simulink model "MobileSimulator"  (R2020a)
settings: Solver=FixedStepAuto  StartTime=0.0  StopTime=5  FixedStep=0.0001  MaxStep=0.1  RelTol=1e-3
undefined symbols (not defined in the file): rad, s
libraries: simulink x7, aerolibconvert2 x4
settings Model: Creator=DELL  LastModifiedBy=DELL

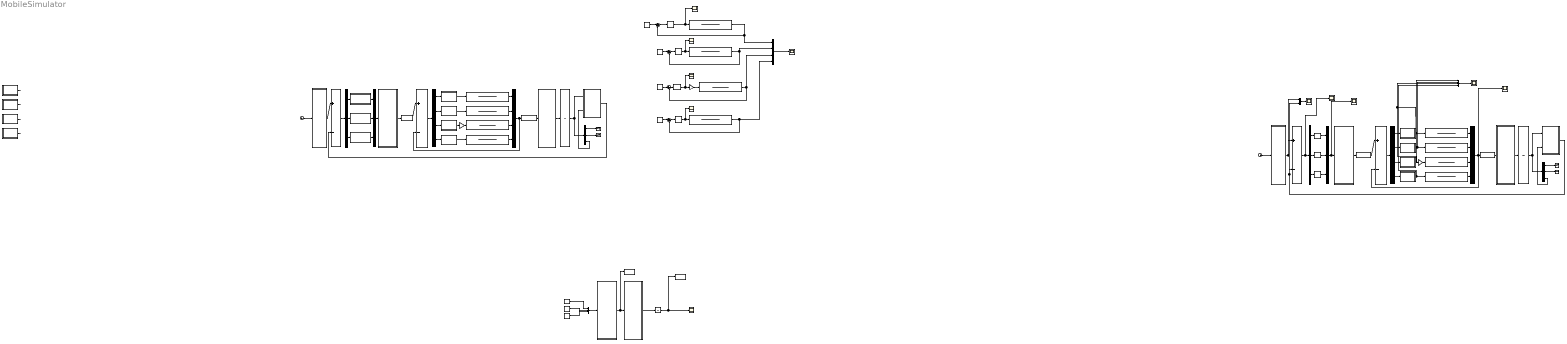
== system MobileSimulator ==
  note: Position Controller
  note: Velocity Controller
  note: Position Controller
  note: Velocity Controller
  Angular Velocity Conversion : aerolibconvert2/Angular Velocity Conversion  IU=rad/s  OU=rpm
  Angular Velocity Conversion1 : aerolibconvert2/Angular Velocity Conversion  IU=rpm  OU=rad/s
  Angular Velocity Conversion2 : aerolibconvert2/Angular Velocity Conversion  IU=rad/s  OU=rpm
  Angular Velocity Conversion3 : aerolibconvert2/Angular Velocity Conversion  IU=rpm  OU=rad/s
  Clock : Clock
  Clock1 : Clock
  Constant{,1..3} (4 alike) : Constant  Value=320
  Constant4 : Constant
  Constant5 : Constant
  Constant6 : Constant  Value=0
  Demux : Demux
  Demux{1,3..4,11} (4 alike) : Demux  Outputs=3
  Demux2 : Demux
  DesiresTrajectory : MATLAB Function  TreatAsAtomicUnit=on
  DesiresTrajectory1 : MATLAB Function  TreatAsAtomicUnit=on
  DriverMotor_1 : TransferFcn  Numerator=[6226000]  Denominator=[1 17030 178900]
  DriverMotor_10 : TransferFcn  Numerator=[6500000]  Denominator=[1 17520 180300]
  DriverMotor_11 : TransferFcn  Numerator=[1081000]  Denominator=[1 4692 40510]
  DriverMotor_12 : TransferFcn  Numerator=[7418000]  Denominator=[1 19890 214900]
  DriverMotor_2 : TransferFcn  Numerator=[6500000]  Denominator=[1 17520 180300]
  DriverMotor_3 : TransferFcn  Numerator=[1081000]  Denominator=[1 4692 40510]
  DriverMotor_4 : TransferFcn  Numerator=[7418000]  Denominator=[1 19890 214900]
  DriverMotor_5 : TransferFcn  Numerator=[6500000]  Denominator=[1 17520 180300]
  DriverMotor_6 : TransferFcn  Numerator=[6226000]  Denominator=[1 17030 178900]
  DriverMotor_7 : TransferFcn  Numerator=[1081000]  Denominator=[1 4692 40510]
  DriverMotor_8 : TransferFcn  Numerator=[7418000]  Denominator=[1 19890 214900]
  DriverMotor_9 : TransferFcn  Numerator=[6226000]  Denominator=[1 17030 178900]
  ForwardKinematic : MATLAB Function  TreatAsAtomicUnit=on
  ForwardKinematic1 : MATLAB Function  TreatAsAtomicUnit=on
  ForwardKinematic2 : MATLAB Function  TreatAsAtomicUnit=on
  Gain1 : Gain  Gain=1.3
  Gain2 : Gain  Gain=1.3
  Gain3 : Gain  Gain=1.3
  Integral : Integrator
  Integral1 : Integrator
  Integrator : Integrator
  InverseKinematics1 : MATLAB Function  TreatAsAtomicUnit=on
  InverseKinematics2 : MATLAB Function  TreatAsAtomicUnit=on
  InverseKinematics3 : MATLAB Function  TreatAsAtomicUnit=on
  Mux{,1,4,12} (4 alike) : Mux
  Mux2 : Mux  Inputs=3
  Mux3 : Mux  Inputs=3
  Mux5 : Mux  Inputs=3
  Mux6 : Mux  Inputs=2
  PDTheta : Subsystem
  PDX : Subsystem
  PDY : Subsystem
  PID Controller10 : simulink/Continuous/PID Controller  Controller=PI  Form=Parallel  TimeDomain=Continuous-time  UseExternalTs=off  SampleTime=-1  IntegratorMethod=Forward Euler  FilterMethod=Forward Euler  ControllerParametersSource=internal  P=0.460464335792483  I=15.4926513743787  D=0  UseFilter=on  N=100  TunerSelectOption=Transfer Function Based (PID Tuner App)  InitialConditionSource=internal  InitialConditionForIntegrator=0  InitialConditionForFilter=0  DifferentiatorICPrevScaledInput=0  ExternalReset=none  TrackingMode=off  Kt=1  LimitOutput=on  UpperSaturationLimit=24  LowerSaturationLimit=-24  LinearizeAsGain=on  AntiWindupMode=none  Kb=1  POutMin=[]  POutMax=[]  IOutMin=[]  IOutMax=[]  DOutMin=[]  DOutMax=[]  NOutMin=[]  NOutMax=[]  SumOutMin=[]  SumOutMax=[]  SaturationOutMin=[]  SaturationOutMax=[]  PParamMin=[]  PParamMax=[]  IParamMin=[]  IParamMax=[]  DParamMin=[]  DParamMax=[]  NParamMin=[]  NParamMax=[]  KbParamMin=[]  KbParamMax=[]  KtParamMin=[]  KtParamMax=[]  KbOutMin=[]  KbOutMax=[]  KtOutMin=[]  KtOutMax=[]  IntegratorOutMin=[]  IntegratorOutMax=[]  FilterOutMin=[]  FilterOutMax=[]  SumI1OutMin=[]  SumI1OutMax=[]  SumI2OutMin=[]  SumI2OutMax=[]  SumI3OutMin=[]  SumI3OutMax=[]  SumI4OutMin=[]  SumI4OutMax=[]  SumDOutMin=[]  SumDOutMax=[]  DifferentiatorOutMin=[]  DifferentiatorOutMax=[]  FilterDiffOutCoefMin=[]  FilterDiffOutCoefMax=[]  ReciprocalOutMin=[]  ReciprocalOutMax=[]  SumDenOutMin=[]  SumDenOutMax=[]  SumNumOutMin=[]  SumNumOutMax=[]  DivideOutMin=[]  DivideOutMax=[]  UdiffTsProdOutMin=[]  UdiffTsProdOutMax=[]  NTsProdOutMin=[]  NTsProdOutMax=[]  UintegralTsProdOutMin=[]  UintegralTsProdOutMax=[]  UngainTsProdOutMin=[]  UngainTsProdOutMax=[]  IntegratorContinuousStateAttributes=''  IntegratorStateMustResolveToSignalObject=off  IntegratorRTWStateStorageClass=Auto  FilterContinuousStateAttributes=''  FilterStateMustResolveToSignalObject=off  FilterRTWStateStorageClass=Auto  ParallelPVariant=InternalParameters  IdealPVariant=Disabled  IVariant=InternalParameters  DVariant=Disabled  IntegratorVariant=Continuous  SatVariant=Enabled  AWVariant=Passthrough  PCopyVariant=Disabled  TRVariant=Disabled  FdbkBlocksVariant=Forward  IdealPFdbkVariant=Disabled  SatFdbkVariant=Disabled  DerivativeFilterVariant=Disabled  NVariant=Disabled  NCopyVariant=Disabled_SignalSpec  FilterICVariant=Disabled  IntegratorICVariant=InternalICs  ExternalResetVariant=Disabled  TRSumVariant=Passthrough  SumFdbkVariant=Disabled  SumVariant=Sum_PI  TsampFilterVariant=InternalTs  TsampNgainVariant=Passthrough  TsampIntegralVariant=Passthrough
  PID Controller4 : simulink/Continuous/PID Controller  Controller=PD  Form=Parallel  TimeDomain=Continuous-time  UseExternalTs=off  SampleTime=-1  IntegratorMethod=Forward Euler  FilterMethod=Forward Euler  ControllerParametersSource=internal  P=31.494456693384  I=1403.5644395001  D=0  UseFilter=on  N=100  TunerSelectOption=Transfer Function Based (PID Tuner App)  InitialConditionSource=internal  InitialConditionForIntegrator=0  InitialConditionForFilter=0  DifferentiatorICPrevScaledInput=0  ExternalReset=none  TrackingMode=off  Kt=1  LimitOutput=on  UpperSaturationLimit=1  LowerSaturationLimit=-1  LinearizeAsGain=on  AntiWindupMode=none  Kb=1  POutMin=[]  POutMax=[]  IOutMin=[]  IOutMax=[]  DOutMin=[]  DOutMax=[]  NOutMin=[]  NOutMax=[]  SumOutMin=[]  SumOutMax=[]  SaturationOutMin=[]  SaturationOutMax=[]  PParamMin=[]  PParamMax=[]  IParamMin=[]  IParamMax=[]  DParamMin=[]  DParamMax=[]  NParamMin=[]  NParamMax=[]  KbParamMin=[]  KbParamMax=[]  KtParamMin=[]  KtParamMax=[]  KbOutMin=[]  KbOutMax=[]  KtOutMin=[]  KtOutMax=[]  IntegratorOutMin=[]  IntegratorOutMax=[]  FilterOutMin=[]  FilterOutMax=[]  SumI1OutMin=[]  SumI1OutMax=[]  SumI2OutMin=[]  SumI2OutMax=[]  SumI3OutMin=[]  SumI3OutMax=[]  SumI4OutMin=[]  SumI4OutMax=[]  SumDOutMin=[]  SumDOutMax=[]  DifferentiatorOutMin=[]  DifferentiatorOutMax=[]  FilterDiffOutCoefMin=[]  FilterDiffOutCoefMax=[]  ReciprocalOutMin=[]  ReciprocalOutMax=[]  SumDenOutMin=[]  SumDenOutMax=[]  SumNumOutMin=[]  SumNumOutMax=[]  DivideOutMin=[]  DivideOutMax=[]  UdiffTsProdOutMin=[]  UdiffTsProdOutMax=[]  NTsProdOutMin=[]  NTsProdOutMax=[]  UintegralTsProdOutMin=[]  UintegralTsProdOutMax=[]  UngainTsProdOutMin=[]  UngainTsProdOutMax=[]  IntegratorContinuousStateAttributes=''  IntegratorStateMustResolveToSignalObject=off  IntegratorRTWStateStorageClass=Auto  FilterContinuousStateAttributes=''  FilterStateMustResolveToSignalObject=off  FilterRTWStateStorageClass=Auto  ParallelPVariant=InternalParameters  IdealPVariant=Disabled  IVariant=Disabled  DVariant=InternalParameters  IntegratorVariant=Disabled  SatVariant=Enabled  AWVariant=Disabled  PCopyVariant=Disabled  TRVariant=Disabled  FdbkBlocksVariant=Forward  IdealPFdbkVariant=Disabled  SatFdbkVariant=Disabled  DerivativeFilterVariant=ContFilter  NVariant=InternalParameters  NCopyVariant=Disabled  FilterICVariant=InternalICsFilter  IntegratorICVariant=Disabled  ExternalResetVariant=Disabled  TRSumVariant=Passthrough  SumFdbkVariant=Disabled  SumVariant=Sum_PD  TsampFilterVariant=InternalTs  TsampNgainVariant=Passthrough  TsampIntegralVariant=Disabled_SignalSpec
  PID Controller5 : simulink/Continuous/PID Controller  Controller=PD  Form=Parallel  TimeDomain=Continuous-time  UseExternalTs=off  SampleTime=-1  IntegratorMethod=Forward Euler  FilterMethod=Forward Euler  ControllerParametersSource=internal  P=12.3118231803941  I=1  D=0  UseFilter=on  N=100  TunerSelectOption=Transfer Function Based (PID Tuner App)  InitialConditionSource=internal  InitialConditionForIntegrator=0  InitialConditionForFilter=0  DifferentiatorICPrevScaledInput=0  ExternalReset=none  TrackingMode=off  Kt=1  LimitOutput=on  UpperSaturationLimit=1  LowerSaturationLimit=-1  LinearizeAsGain=off  AntiWindupMode=none  Kb=1  POutMin=[]  POutMax=[]  IOutMin=[]  IOutMax=[]  DOutMin=[]  DOutMax=[]  NOutMin=[]  NOutMax=[]  SumOutMin=[]  SumOutMax=[]  SaturationOutMin=[]  SaturationOutMax=[]  PParamMin=[]  PParamMax=[]  IParamMin=[]  IParamMax=[]  DParamMin=[]  DParamMax=[]  NParamMin=[]  NParamMax=[]  KbParamMin=[]  KbParamMax=[]  KtParamMin=[]  KtParamMax=[]  KbOutMin=[]  KbOutMax=[]  KtOutMin=[]  KtOutMax=[]  IntegratorOutMin=[]  IntegratorOutMax=[]  FilterOutMin=[]  FilterOutMax=[]  SumI1OutMin=[]  SumI1OutMax=[]  SumI2OutMin=[]  SumI2OutMax=[]  SumI3OutMin=[]  SumI3OutMax=[]  SumI4OutMin=[]  SumI4OutMax=[]  SumDOutMin=[]  SumDOutMax=[]  DifferentiatorOutMin=[]  DifferentiatorOutMax=[]  FilterDiffOutCoefMin=[]  FilterDiffOutCoefMax=[]  ReciprocalOutMin=[]  ReciprocalOutMax=[]  SumDenOutMin=[]  SumDenOutMax=[]  SumNumOutMin=[]  SumNumOutMax=[]  DivideOutMin=[]  DivideOutMax=[]  UdiffTsProdOutMin=[]  UdiffTsProdOutMax=[]  NTsProdOutMin=[]  NTsProdOutMax=[]  UintegralTsProdOutMin=[]  UintegralTsProdOutMax=[]  UngainTsProdOutMin=[]  UngainTsProdOutMax=[]  IntegratorContinuousStateAttributes=''  IntegratorStateMustResolveToSignalObject=off  IntegratorRTWStateStorageClass=Auto  FilterContinuousStateAttributes=''  FilterStateMustResolveToSignalObject=off  FilterRTWStateStorageClass=Auto  ParallelPVariant=InternalParameters  IdealPVariant=Disabled  IVariant=Disabled  DVariant=InternalParameters  IntegratorVariant=Disabled  SatVariant=Enabled  AWVariant=Disabled  PCopyVariant=Disabled  TRVariant=Disabled  FdbkBlocksVariant=Forward  IdealPFdbkVariant=Disabled  SatFdbkVariant=Disabled  DerivativeFilterVariant=ContFilter  NVariant=InternalParameters  NCopyVariant=Disabled  FilterICVariant=InternalICsFilter  IntegratorICVariant=Disabled  ExternalResetVariant=Disabled  TRSumVariant=Passthrough  SumFdbkVariant=Disabled  SumVariant=Sum_PD  TsampFilterVariant=InternalTs  TsampNgainVariant=Passthrough  TsampIntegralVariant=Disabled_SignalSpec
  PID Controller6 : simulink/Continuous/PID Controller  Controller=PD  Form=Parallel  TimeDomain=Continuous-time  UseExternalTs=off  SampleTime=-1  IntegratorMethod=Forward Euler  FilterMethod=Forward Euler  ControllerParametersSource=internal  P=17.283663240322  I=1  D=0  UseFilter=on  N=100  TunerSelectOption=Transfer Function Based (PID Tuner App)  InitialConditionSource=internal  InitialConditionForIntegrator=0  InitialConditionForFilter=0  DifferentiatorICPrevScaledInput=0  ExternalReset=none  TrackingMode=off  Kt=1  LimitOutput=on  UpperSaturationLimit=1  LowerSaturationLimit=-1  LinearizeAsGain=on  AntiWindupMode=none  Kb=1  POutMin=[]  POutMax=[]  IOutMin=[]  IOutMax=[]  DOutMin=[]  DOutMax=[]  NOutMin=[]  NOutMax=[]  SumOutMin=[]  SumOutMax=[]  SaturationOutMin=[]  SaturationOutMax=[]  PParamMin=[]  PParamMax=[]  IParamMin=[]  IParamMax=[]  DParamMin=[]  DParamMax=[]  NParamMin=[]  NParamMax=[]  KbParamMin=[]  KbParamMax=[]  KtParamMin=[]  KtParamMax=[]  KbOutMin=[]  KbOutMax=[]  KtOutMin=[]  KtOutMax=[]  IntegratorOutMin=[]  IntegratorOutMax=[]  FilterOutMin=[]  FilterOutMax=[]  SumI1OutMin=[]  SumI1OutMax=[]  SumI2OutMin=[]  SumI2OutMax=[]  SumI3OutMin=[]  SumI3OutMax=[]  SumI4OutMin=[]  SumI4OutMax=[]  SumDOutMin=[]  SumDOutMax=[]  DifferentiatorOutMin=[]  DifferentiatorOutMax=[]  FilterDiffOutCoefMin=[]  FilterDiffOutCoefMax=[]  ReciprocalOutMin=[]  ReciprocalOutMax=[]  SumDenOutMin=[]  SumDenOutMax=[]  SumNumOutMin=[]  SumNumOutMax=[]  DivideOutMin=[]  DivideOutMax=[]  UdiffTsProdOutMin=[]  UdiffTsProdOutMax=[]  NTsProdOutMin=[]  NTsProdOutMax=[]  UintegralTsProdOutMin=[]  UintegralTsProdOutMax=[]  UngainTsProdOutMin=[]  UngainTsProdOutMax=[]  IntegratorContinuousStateAttributes=''  IntegratorStateMustResolveToSignalObject=off  IntegratorRTWStateStorageClass=Auto  FilterContinuousStateAttributes=''  FilterStateMustResolveToSignalObject=off  FilterRTWStateStorageClass=Auto  ParallelPVariant=InternalParameters  IdealPVariant=Disabled  IVariant=Disabled  DVariant=InternalParameters  IntegratorVariant=Disabled  SatVariant=Enabled  AWVariant=Disabled  PCopyVariant=Disabled  TRVariant=Disabled  FdbkBlocksVariant=Forward  IdealPFdbkVariant=Disabled  SatFdbkVariant=Disabled  DerivativeFilterVariant=ContFilter  NVariant=InternalParameters  NCopyVariant=Disabled  FilterICVariant=InternalICsFilter  IntegratorICVariant=Disabled  ExternalResetVariant=Disabled  TRSumVariant=Passthrough  SumFdbkVariant=Disabled  SumVariant=Sum_PD  TsampFilterVariant=InternalTs  TsampNgainVariant=Passthrough  TsampIntegralVariant=Disabled_SignalSpec
  PID Controller7 : simulink/Continuous/PID Controller  Controller=PI  Form=Parallel  TimeDomain=Continuous-time  UseExternalTs=off  SampleTime=-1  IntegratorMethod=Forward Euler  FilterMethod=Forward Euler  ControllerParametersSource=internal  P=0.460464335792483  I=15.4926513743787  D=0  UseFilter=on  N=100  TunerSelectOption=Transfer Function Based (PID Tuner App)  InitialConditionSource=internal  InitialConditionForIntegrator=0  InitialConditionForFilter=0  DifferentiatorICPrevScaledInput=0  ExternalReset=none  TrackingMode=off  Kt=1  LimitOutput=on  UpperSaturationLimit=24  LowerSaturationLimit=-24  LinearizeAsGain=on  AntiWindupMode=none  Kb=1  POutMin=[]  POutMax=[]  IOutMin=[]  IOutMax=[]  DOutMin=[]  DOutMax=[]  NOutMin=[]  NOutMax=[]  SumOutMin=[]  SumOutMax=[]  SaturationOutMin=[]  SaturationOutMax=[]  PParamMin=[]  PParamMax=[]  IParamMin=[]  IParamMax=[]  DParamMin=[]  DParamMax=[]  NParamMin=[]  NParamMax=[]  KbParamMin=[]  KbParamMax=[]  KtParamMin=[]  KtParamMax=[]  KbOutMin=[]  KbOutMax=[]  KtOutMin=[]  KtOutMax=[]  IntegratorOutMin=[]  IntegratorOutMax=[]  FilterOutMin=[]  FilterOutMax=[]  SumI1OutMin=[]  SumI1OutMax=[]  SumI2OutMin=[]  SumI2OutMax=[]  SumI3OutMin=[]  SumI3OutMax=[]  SumI4OutMin=[]  SumI4OutMax=[]  SumDOutMin=[]  SumDOutMax=[]  DifferentiatorOutMin=[]  DifferentiatorOutMax=[]  FilterDiffOutCoefMin=[]  FilterDiffOutCoefMax=[]  ReciprocalOutMin=[]  ReciprocalOutMax=[]  SumDenOutMin=[]  SumDenOutMax=[]  SumNumOutMin=[]  SumNumOutMax=[]  DivideOutMin=[]  DivideOutMax=[]  UdiffTsProdOutMin=[]  UdiffTsProdOutMax=[]  NTsProdOutMin=[]  NTsProdOutMax=[]  UintegralTsProdOutMin=[]  UintegralTsProdOutMax=[]  UngainTsProdOutMin=[]  UngainTsProdOutMax=[]  IntegratorContinuousStateAttributes=''  IntegratorStateMustResolveToSignalObject=off  IntegratorRTWStateStorageClass=Auto  FilterContinuousStateAttributes=''  FilterStateMustResolveToSignalObject=off  FilterRTWStateStorageClass=Auto  ParallelPVariant=InternalParameters  IdealPVariant=Disabled  IVariant=InternalParameters  DVariant=Disabled  IntegratorVariant=Continuous  SatVariant=Enabled  AWVariant=Passthrough  PCopyVariant=Disabled  TRVariant=Disabled  FdbkBlocksVariant=Forward  IdealPFdbkVariant=Disabled  SatFdbkVariant=Disabled  DerivativeFilterVariant=Disabled  NVariant=Disabled  NCopyVariant=Disabled_SignalSpec  FilterICVariant=Disabled  IntegratorICVariant=InternalICs  ExternalResetVariant=Disabled  TRSumVariant=Passthrough  SumFdbkVariant=Disabled  SumVariant=Sum_PI  TsampFilterVariant=InternalTs  TsampNgainVariant=Passthrough  TsampIntegralVariant=Passthrough
  PID Controller8 : simulink/Continuous/PID Controller  Controller=PI  Form=Parallel  TimeDomain=Continuous-time  UseExternalTs=off  SampleTime=-1  IntegratorMethod=Forward Euler  FilterMethod=Forward Euler  ControllerParametersSource=internal  P=0.460464335792483  I=15.4926513743787  D=0  UseFilter=on  N=100  TunerSelectOption=Transfer Function Based (PID Tuner App)  InitialConditionSource=internal  InitialConditionForIntegrator=0  InitialConditionForFilter=0  DifferentiatorICPrevScaledInput=0  ExternalReset=none  TrackingMode=off  Kt=1  LimitOutput=on  UpperSaturationLimit=24  LowerSaturationLimit=-24  LinearizeAsGain=on  AntiWindupMode=none  Kb=1  POutMin=[]  POutMax=[]  IOutMin=[]  IOutMax=[]  DOutMin=[]  DOutMax=[]  NOutMin=[]  NOutMax=[]  SumOutMin=[]  SumOutMax=[]  SaturationOutMin=[]  SaturationOutMax=[]  PParamMin=[]  PParamMax=[]  IParamMin=[]  IParamMax=[]  DParamMin=[]  DParamMax=[]  NParamMin=[]  NParamMax=[]  KbParamMin=[]  KbParamMax=[]  KtParamMin=[]  KtParamMax=[]  KbOutMin=[]  KbOutMax=[]  KtOutMin=[]  KtOutMax=[]  IntegratorOutMin=[]  IntegratorOutMax=[]  FilterOutMin=[]  FilterOutMax=[]  SumI1OutMin=[]  SumI1OutMax=[]  SumI2OutMin=[]  SumI2OutMax=[]  SumI3OutMin=[]  SumI3OutMax=[]  SumI4OutMin=[]  SumI4OutMax=[]  SumDOutMin=[]  SumDOutMax=[]  DifferentiatorOutMin=[]  DifferentiatorOutMax=[]  FilterDiffOutCoefMin=[]  FilterDiffOutCoefMax=[]  ReciprocalOutMin=[]  ReciprocalOutMax=[]  SumDenOutMin=[]  SumDenOutMax=[]  SumNumOutMin=[]  SumNumOutMax=[]  DivideOutMin=[]  DivideOutMax=[]  UdiffTsProdOutMin=[]  UdiffTsProdOutMax=[]  NTsProdOutMin=[]  NTsProdOutMax=[]  UintegralTsProdOutMin=[]  UintegralTsProdOutMax=[]  UngainTsProdOutMin=[]  UngainTsProdOutMax=[]  IntegratorContinuousStateAttributes=''  IntegratorStateMustResolveToSignalObject=off  IntegratorRTWStateStorageClass=Auto  FilterContinuousStateAttributes=''  FilterStateMustResolveToSignalObject=off  FilterRTWStateStorageClass=Auto  ParallelPVariant=InternalParameters  IdealPVariant=Disabled  IVariant=InternalParameters  DVariant=Disabled  IntegratorVariant=Continuous  SatVariant=Enabled  AWVariant=Passthrough  PCopyVariant=Disabled  TRVariant=Disabled  FdbkBlocksVariant=Forward  IdealPFdbkVariant=Disabled  SatFdbkVariant=Disabled  DerivativeFilterVariant=Disabled  NVariant=Disabled  NCopyVariant=Disabled_SignalSpec  FilterICVariant=Disabled  IntegratorICVariant=InternalICs  ExternalResetVariant=Disabled  TRSumVariant=Passthrough  SumFdbkVariant=Disabled  SumVariant=Sum_PI  TsampFilterVariant=InternalTs  TsampNgainVariant=Passthrough  TsampIntegralVariant=Passthrough
  PID Controller9 : simulink/Continuous/PID Controller  Controller=PI  Form=Parallel  TimeDomain=Continuous-time  UseExternalTs=off  SampleTime=-1  IntegratorMethod=Forward Euler  FilterMethod=Forward Euler  ControllerParametersSource=internal  P=0.537194587615843  I=14.0924173229999  D=0  UseFilter=on  N=100  TunerSelectOption=Transfer Function Based (PID Tuner App)  InitialConditionSource=internal  InitialConditionForIntegrator=0  InitialConditionForFilter=0  DifferentiatorICPrevScaledInput=0  ExternalReset=none  TrackingMode=off  Kt=1  LimitOutput=on  UpperSaturationLimit=24  LowerSaturationLimit=-24  LinearizeAsGain=on  AntiWindupMode=none  Kb=1  POutMin=[]  POutMax=[]  IOutMin=[]  IOutMax=[]  DOutMin=[]  DOutMax=[]  NOutMin=[]  NOutMax=[]  SumOutMin=[]  SumOutMax=[]  SaturationOutMin=[]  SaturationOutMax=[]  PParamMin=[]  PParamMax=[]  IParamMin=[]  IParamMax=[]  DParamMin=[]  DParamMax=[]  NParamMin=[]  NParamMax=[]  KbParamMin=[]  KbParamMax=[]  KtParamMin=[]  KtParamMax=[]  KbOutMin=[]  KbOutMax=[]  KtOutMin=[]  KtOutMax=[]  IntegratorOutMin=[]  IntegratorOutMax=[]  FilterOutMin=[]  FilterOutMax=[]  SumI1OutMin=[]  SumI1OutMax=[]  SumI2OutMin=[]  SumI2OutMax=[]  SumI3OutMin=[]  SumI3OutMax=[]  SumI4OutMin=[]  SumI4OutMax=[]  SumDOutMin=[]  SumDOutMax=[]  DifferentiatorOutMin=[]  DifferentiatorOutMax=[]  FilterDiffOutCoefMin=[]  FilterDiffOutCoefMax=[]  ReciprocalOutMin=[]  ReciprocalOutMax=[]  SumDenOutMin=[]  SumDenOutMax=[]  SumNumOutMin=[]  SumNumOutMax=[]  DivideOutMin=[]  DivideOutMax=[]  UdiffTsProdOutMin=[]  UdiffTsProdOutMax=[]  NTsProdOutMin=[]  NTsProdOutMax=[]  UintegralTsProdOutMin=[]  UintegralTsProdOutMax=[]  UngainTsProdOutMin=[]  UngainTsProdOutMax=[]  IntegratorContinuousStateAttributes=''  IntegratorStateMustResolveToSignalObject=off  IntegratorRTWStateStorageClass=Auto  FilterContinuousStateAttributes=''  FilterStateMustResolveToSignalObject=off  FilterRTWStateStorageClass=Auto  ParallelPVariant=InternalParameters  IdealPVariant=Disabled  IVariant=InternalParameters  DVariant=Disabled  IntegratorVariant=Continuous  SatVariant=Enabled  AWVariant=Passthrough  PCopyVariant=Disabled  TRVariant=Disabled  FdbkBlocksVariant=Forward  IdealPFdbkVariant=Disabled  SatFdbkVariant=Disabled  DerivativeFilterVariant=Disabled  NVariant=Disabled  NCopyVariant=Disabled_SignalSpec  FilterICVariant=Disabled  IntegratorICVariant=InternalICs  ExternalResetVariant=Disabled  TRSumVariant=Passthrough  SumFdbkVariant=Disabled  SumVariant=Sum_PI  TsampFilterVariant=InternalTs  TsampNgainVariant=Passthrough  TsampIntegralVariant=Passthrough
  PI_Motor_1. : Subsystem
  PI_Motor_10 : Subsystem
  PI_Motor_11 : Subsystem
  PI_Motor_12 : Subsystem
  PI_Motor_2. : Subsystem
  PI_Motor_3. : Subsystem
  PI_Motor_4. : Subsystem
  PI_Motor_5 : Subsystem
  PI_Motor_6 : Subsystem
  PI_Motor_7 : Subsystem
  PI_Motor_8 : Subsystem
  PI_Motor_9 : Subsystem
  Scope{,2..3,6..8,11,13..15,17} (11 alike) : Scope
  Sum{,1,3..6} (6 alike) : Sum  Inputs=|+-
  Sum. : Sum  Inputs=|+-
  Sum.1 : Sum  Inputs=|+-
  Terminator{1..2,6..7} (4 alike) : Terminator
  To File : ToFile  Filename=D:\Documents\DOAN\DO-AN\matlab\datamat\dothi\banhxe.mat
  To File1 : ToFile  Filename=D:\Documents\DOAN\DO-AN\matlab\datamat\dothi\vitri.mat
  ToGlobal : MATLAB Function  TreatAsAtomicUnit=on
  ToGlobal1 : MATLAB Function  TreatAsAtomicUnit=on
  wires:
  PI_Motor_1./1(signal) -> DriverMotor_1/1
  PI_Motor_2./1(signal) -> DriverMotor_2/1
  PI_Motor_4./1(signal) -> DriverMotor_4/1
  DriverMotor_1/1 -> Mux/1
  DriverMotor_2/1 -> Mux/2
  DriverMotor_4/1 -> Mux/4
  Demux/1 -> PI_Motor_1./1(error)
  Demux/2 -> PI_Motor_2./1(error)
  Demux/4 -> PI_Motor_4./1(error)
  Demux/3 -> PI_Motor_3./1(error)
  Sum/1 -> Demux/1
  InverseKinematics2/1(w) -> Angular Velocity Conversion/1
  ForwardKinematic/1(q_dot_r) -> Integral/1
  Sum./1 -> Demux1/1
  Integral/1 -> Demux11/1, ToGlobal/1(q_r)
  Demux11/1 -> Terminator6/1
  Demux11/2 -> Terminator7/1
  ToGlobal/1(q) -> Sum./2
  DesiresTrajectory/1(q) -> Sum./1
  Clock/1 -> DesiresTrajectory/1(t)
  Mux2/1 -> InverseKinematics2/1(q_dot_r)
  Demux11/3 -> ToGlobal/2(theta)
  Demux1/1 -> PDX/1(error)
  PDX/1(signal) -> Mux2/1
  Demux1/2 -> PDY/1(error)
  PDY/1(signal) -> Mux2/2
  Demux1/3 -> PDTheta/1(error)
  PDTheta/1(signal) -> Mux2/3
  Mux/1 -> Sum/2, Angular Velocity Conversion1/1
  Angular Velocity Conversion/1 -> Sum/1
  Angular Velocity Conversion1/1 -> ForwardKinematic/1(w)
  PID Controller8/1 -> Scope11/1, DriverMotor_5/1
  Sum3/1 -> PID Controller8/1
  PI_Motor_5/1(signal) -> ?
  PI_Motor_6/1(signal) -> ?
  PI_Motor_8/1(signal) -> ?
  PI_Motor_7/1(signal) -> ?
  Sum4/1 -> PID Controller7/1
  Constant3/1 -> Sum4/1
  Constant/1 -> Sum3/1
  DriverMotor_5/1 -> Mux12/2, Sum3/2
  PID Controller7/1 -> DriverMotor_6/1, Scope13/1
  DriverMotor_6/1 -> Sum4/2, Mux12/1
  Sum5/1 -> PID Controller9/1
  Constant1/1 -> Sum5/1
  Sum6/1 -> PID Controller10/1
  PID Controller10/1 -> DriverMotor_8/1, Scope17/1
  DriverMotor_8/1 -> Mux12/4, Sum6/2
  Constant2/1 -> Sum6/1
  DriverMotor_7/1 -> Mux12/3, Sum5/2
  Mux12/1 -> Scope14/1
  DriverMotor_3/1 -> Mux/3
  PID Controller9/1 -> Gain3/1, Scope15/1
  Gain1/1 -> DriverMotor_3/1
  Gain3/1 -> DriverMotor_7/1
  DriverMotor_12/1 -> Mux1/4
  Demux4/1 -> Terminator1/1
  PI_Motor_11/1(signal) -> DriverMotor_9/1, Mux4/1
  DriverMotor_10/1 -> Mux1/2
  Angular Velocity Conversion3/1 -> ForwardKinematic1/1(w)
  Demux3/2 -> PID Controller5/1
  Demux3/1 -> PID Controller4/1
  Demux3/3 -> PID Controller6/1
  PID Controller6/1 -> Mux5/3
  Mux6/1 -> Scope2/1
  Demux4/3 -> ToGlobal1/2(theta)
  PID Controller5/1 -> Mux5/2
  ToGlobal1/1(q) -> Mux6/2, Sum.1/2
  Mux5/1 -> InverseKinematics1/1(q_dot_r), Scope6/1
  Demux4/2 -> Terminator2/1
  Demux2/4 -> PI_Motor_9/1(error)
  PI_Motor_9/1(signal) -> DriverMotor_12/1, Mux4/4
  InverseKinematics1/1(w) -> Angular Velocity Conversion2/1
  Integral1/1 -> Demux4/1, ToGlobal1/1(q_r)
  Sum.1/1 -> Scope8/1, Demux3/1
  ForwardKinematic1/1(q_dot_r) -> Integral1/1
  PI_Motor_10/1(signal) -> Mux4/3, Gain2/1
  Sum1/1 -> Demux2/1
  DriverMotor_11/1 -> Mux1/3
  PI_Motor_12/1(signal) -> Mux4/2, DriverMotor_10/1
  Angular Velocity Conversion2/1 -> Sum1/1
  DriverMotor_9/1 -> Mux1/1
  Demux2/2 -> PI_Motor_12/1(error)
  DesiresTrajectory1/1(q) -> Mux6/1, Sum.1/1
  Mux4/1 -> Scope3/1
  Demux2/1 -> PI_Motor_11/1(error)
  PID Controller4/1 -> Mux5/1
  Clock1/1 -> DesiresTrajectory1/1(t)
  Gain2/1 -> DriverMotor_11/1
  Demux2/3 -> PI_Motor_10/1(error)
  Mux1/1 -> Sum1/2, Angular Velocity Conversion3/1, Scope7/1
  PI_Motor_3./1(signal) -> Gain1/1
  InverseKinematics3/1(w) -> To File/1, ForwardKinematic2/1(w)
  Mux3/1 -> InverseKinematics3/1(q_dot_r)
  Constant5/1 -> Mux3/2
  Constant4/1 -> Mux3/1
  Constant6/1 -> Mux3/3
  ForwardKinematic2/1(q_dot_r) -> Integrator/1
  Integrator/1 -> To File1/1, Scope/1

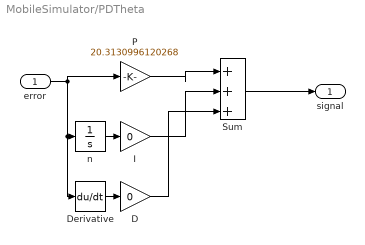
== system MobileSimulator/PDTheta ==
  error : Inport
  D : Gain  Gain=0
  Derivative : Derivative
  I : Gain  Gain=0
  P : Gain  Gain=20.3130996120268
  Sum : Sum  Inputs=|+++
  n : Integrator
  signal : Outport
  wires:
  Derivative/1 -> D/1
  n/1 -> I/1
  I/1 -> Sum/2
  error/1 -> Derivative/1, n/1, P/1
  Sum/1 -> signal/1
  P/1 -> Sum/1
  D/1 -> Sum/3

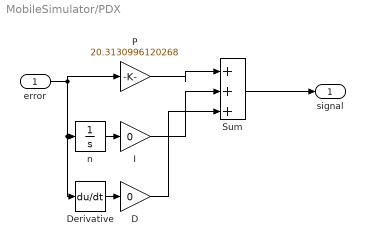
== system MobileSimulator/PDX ==
  error : Inport
  D : Gain  Gain=0
  Derivative : Derivative
  I : Gain  Gain=0
  P : Gain  Gain=20.3130996120268
  Sum : Sum  Inputs=|+++
  n : Integrator
  signal : Outport
  wires:
  Derivative/1 -> D/1
  n/1 -> I/1
  I/1 -> Sum/2
  error/1 -> Derivative/1, n/1, P/1
  Sum/1 -> signal/1
  P/1 -> Sum/1
  D/1 -> Sum/3

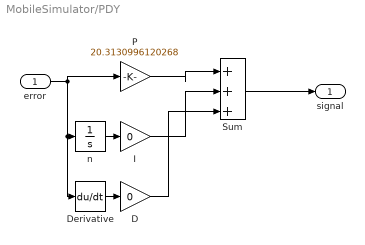
== system MobileSimulator/PDY ==
  error : Inport
  D : Gain  Gain=0
  Derivative : Derivative
  I : Gain  Gain=0
  P : Gain  Gain=20.3130996120268
  Sum : Sum  Inputs=|+++
  n : Integrator
  signal : Outport
  wires:
  Derivative/1 -> D/1
  n/1 -> I/1
  I/1 -> Sum/2
  error/1 -> Derivative/1, n/1, P/1
  Sum/1 -> signal/1
  P/1 -> Sum/1
  D/1 -> Sum/3

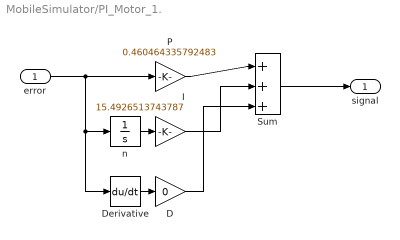
== system MobileSimulator/PI_Motor_1. ==
  error : Inport
  D : Gain  Gain=0
  Derivative : Derivative
  I : Gain  Gain=15.4926513743787
  P : Gain  Gain=0.460464335792483
  Sum : Sum  Inputs=|+++
  n : Integrator
  signal : Outport
  wires:
  error/1 -> P/1, n/1, Derivative/1
  n/1 -> I/1
  P/1 -> Sum/1
  I/1 -> Sum/2
  Derivative/1 -> D/1
  Sum/1 -> signal/1
  D/1 -> Sum/3

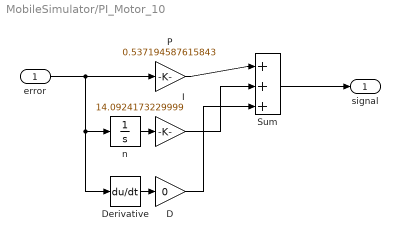
== system MobileSimulator/PI_Motor_10 ==
  error : Inport
  D : Gain  Gain=0
  Derivative : Derivative
  I : Gain  Gain=14.0924173229999
  P : Gain  Gain=0.537194587615843
  Sum : Sum  Inputs=|+++
  n : Integrator
  signal : Outport
  wires:
  Derivative/1 -> D/1
  n/1 -> I/1
  I/1 -> Sum/2
  error/1 -> P/1, n/1, Derivative/1
  Sum/1 -> signal/1
  P/1 -> Sum/1
  D/1 -> Sum/3

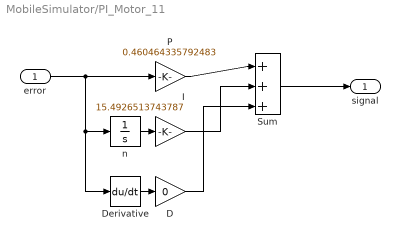
== system MobileSimulator/PI_Motor_11 ==
  error : Inport
  D : Gain  Gain=0
  Derivative : Derivative
  I : Gain  Gain=15.4926513743787
  P : Gain  Gain=0.460464335792483
  Sum : Sum  Inputs=|+++
  n : Integrator
  signal : Outport
  wires:
  error/1 -> P/1, n/1, Derivative/1
  n/1 -> I/1
  P/1 -> Sum/1
  I/1 -> Sum/2
  Derivative/1 -> D/1
  Sum/1 -> signal/1
  D/1 -> Sum/3

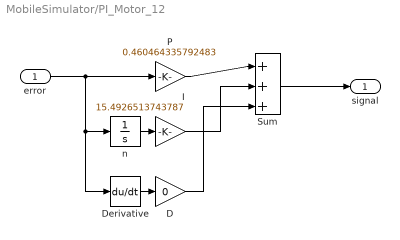
== system MobileSimulator/PI_Motor_12 ==
  error : Inport
  D : Gain  Gain=0
  Derivative : Derivative
  I : Gain  Gain=15.4926513743787
  P : Gain  Gain=0.460464335792483
  Sum : Sum  Inputs=|+++
  n : Integrator
  signal : Outport
  wires:
  error/1 -> P/1, n/1, Derivative/1
  n/1 -> I/1
  P/1 -> Sum/1
  I/1 -> Sum/2
  Derivative/1 -> D/1
  Sum/1 -> signal/1
  D/1 -> Sum/3

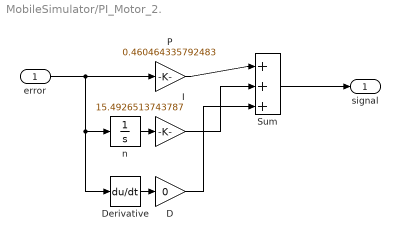
== system MobileSimulator/PI_Motor_2. ==
  error : Inport
  D : Gain  Gain=0
  Derivative : Derivative
  I : Gain  Gain=15.4926513743787
  P : Gain  Gain=0.460464335792483
  Sum : Sum  Inputs=|+++
  n : Integrator
  signal : Outport
  wires:
  error/1 -> P/1, n/1, Derivative/1
  n/1 -> I/1
  P/1 -> Sum/1
  I/1 -> Sum/2
  Derivative/1 -> D/1
  Sum/1 -> signal/1
  D/1 -> Sum/3

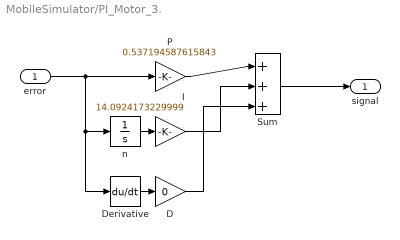
== system MobileSimulator/PI_Motor_3. ==
  error : Inport
  D : Gain  Gain=0
  Derivative : Derivative
  I : Gain  Gain=14.0924173229999
  P : Gain  Gain=0.537194587615843
  Sum : Sum  Inputs=|+++
  n : Integrator
  signal : Outport
  wires:
  Derivative/1 -> D/1
  n/1 -> I/1
  I/1 -> Sum/2
  error/1 -> P/1, n/1, Derivative/1
  Sum/1 -> signal/1
  P/1 -> Sum/1
  D/1 -> Sum/3

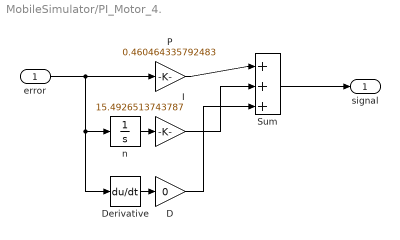
== system MobileSimulator/PI_Motor_4. ==
  error : Inport
  D : Gain  Gain=0
  Derivative : Derivative
  I : Gain  Gain=15.4926513743787
  P : Gain  Gain=0.460464335792483
  Sum : Sum  Inputs=|+++
  n : Integrator
  signal : Outport
  wires:
  error/1 -> P/1, n/1, Derivative/1
  n/1 -> I/1
  P/1 -> Sum/1
  I/1 -> Sum/2
  Derivative/1 -> D/1
  Sum/1 -> signal/1
  D/1 -> Sum/3

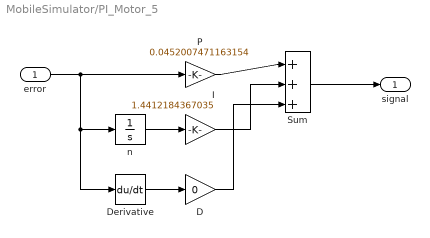
== system MobileSimulator/PI_Motor_5 ==
  error : Inport
  D : Gain  Gain=0
  Derivative : Derivative
  I : Gain  Gain=1.4412184367035
  P : Gain  Gain=0.0452007471163154
  Sum : Sum  Inputs=|+++
  n : Integrator
  signal : Outport
  wires:
  Derivative/1 -> D/1
  n/1 -> I/1
  I/1 -> Sum/2
  error/1 -> P/1, n/1, Derivative/1
  Sum/1 -> signal/1
  P/1 -> Sum/1
  D/1 -> Sum/3

== system MobileSimulator/PI_Motor_6 ==
  error : Inport
  D : Gain  Gain=0
  Derivative : Derivative
  I : Gain  Gain=1.79334556232624
  P : Gain  Gain=0.070850354012992
  Sum : Sum  Inputs=|+++
  n : Integrator
  signal : Outport
  wires:
  Derivative/1 -> D/1
  n/1 -> I/1
  I/1 -> Sum/2
  error/1 -> P/1, n/1, Derivative/1
  Sum/1 -> signal/1
  P/1 -> Sum/1
  D/1 -> Sum/3

== system MobileSimulator/PI_Motor_7 ==
  error : Inport
  D : Gain  Gain=0
  Derivative : Derivative
  I : Gain  Gain=1.79334556232624
  P : Gain  Gain=0.070850354012992
  Sum : Sum  Inputs=|+++
  n : Integrator
  signal : Outport
  wires:
  error/1 -> P/1, n/1, Derivative/1
  n/1 -> I/1
  P/1 -> Sum/1
  I/1 -> Sum/2
  Derivative/1 -> D/1
  Sum/1 -> signal/1
  D/1 -> Sum/3

== system MobileSimulator/PI_Motor_8 ==
  error : Inport
  D : Gain  Gain=0
  Derivative : Derivative
  I : Gain  Gain=1.79334556232624
  P : Gain  Gain=0.070850354012992
  Sum : Sum  Inputs=|+++
  n : Integrator
  signal : Outport
  wires:
  P/1 -> Sum/1
  D/1 -> Sum/3
  Sum/1 -> signal/1
  I/1 -> Sum/2
  n/1 -> I/1
  Derivative/1 -> D/1
  error/1 -> P/1, n/1, Derivative/1

== system MobileSimulator/PI_Motor_9 ==
  error : Inport
  D : Gain  Gain=0
  Derivative : Derivative
  I : Gain  Gain=15.4926513743787
  P : Gain  Gain=0.460464335792483
  Sum : Sum  Inputs=|+++
  n : Integrator
  signal : Outport
  wires:
  error/1 -> P/1, n/1, Derivative/1
  n/1 -> I/1
  P/1 -> Sum/1
  I/1 -> Sum/2
  Derivative/1 -> D/1
  Sum/1 -> signal/1
  D/1 -> Sum/3

== matlab function MobileSimulator/DesiresTrajectory1 ==
  data: t input; q output
function q  = Desired_Trajectory(t)
%Create desires trajectory

% Radius and vecolcity angular
R = 20 ;

% Parametric equation
%x_d = R*sin(t);
%y_d = R*cos(t);

x_d = 0 + 0.5*sin(100*t);
y_d = 0 + 0.5*cos(100*t);

% Derivative of Paramet ric equation
%x_dot_d = R*cos(t);
%y_dot_d = -R*sin(t);
x_dot_d = 0.1;
y_dot_d = 0.1;

theta_d = 0;

% Output
if (x_d >= 5)
    x_d = 5;
    y_d = 5;
end
q = [x_d; y_d; theta_d];

== matlab function MobileSimulator/ForwardKinematic1 ==
  data: w input; q_dot_r output
function q_dot_r = ForwardKinematic(w)

r = 0.03 ; lx = 0.1 ; ly = 0.075 ;

Jacobian_T = (r/4) * [1, 1, 1, 1; -1, 1, 1, -1; -1/(lx + ly), 1/(lx + ly), -1/(lx + ly), 1/(lx + ly)];

q_dot_r = Jacobian_T * w;

== matlab function MobileSimulator/InverseKinematics1 ==
  data: q_dot_r input; w output
function w = Jacobian(q_dot_r)

% This function to calculate velocity angular of wheels basing on linear
% velocity and derivative of rotating angle of mobile platform 


% Configurate of mobile platform
r = 0.05 ; lx = 0.15 ; ly = 0.15 ;
a = 1/r;
Jacobian = a * [1, -1, -(lx + ly); 1, 1, (lx + ly); 1, 1, -(lx + ly); 1, -1, (lx + ly)];

w = Jacobian * q_dot_r;
% Output

== matlab function MobileSimulator/ToGlobal1 ==
  data: q_r input; theta input; q output
function q = Transform(q_r, theta)

% This function to transform global coordinates to mobile platform coordinates

% Transform matrix
R = [cos(theta), -sin(theta), 0; sin(theta), cos(theta), 0; 0, 0, 1];


% Output
q = R * q_r;

== matlab function MobileSimulator/InverseKinematics2 ==
  data: q_dot_r input; w output
function w = Jacobian(q_dot_r)

% This function to calculate velocity angular of wheels basing on linear
% velocity and derivative of rotating angle of mobile platform 


% Configurate of mobile platform
r = 0.05 ; lx = 0.15 ; ly = 0.15 ;
a = 1/r;
Jacobian = a * [1, -1, -(lx + ly); 1, 1, (lx + ly); 1, 1, -(lx + ly); 1, -1, (lx + ly)];

w = Jacobian * q_dot_r;
% Output

== matlab function MobileSimulator/InverseKinematics3 ==
  data: q_dot_r input; w output
function w = Jacobian(q_dot_r)

% This function to calculate velocity angular of wheels basing on linear
% velocity and derivative of rotating angle of mobile platform 


% Configurate of mobile platform
r = 0.05 ; lx = 0.225 ; ly = 0.105;
a = 1/r;
Jacobian = a * [1, 1, -(lx + ly); 1, -1, (lx + ly); 1, 1, (lx + ly); 1, -1, -(lx + ly)];

w = Jacobian * q_dot_r;
% Output

== matlab function MobileSimulator/ForwardKinematic2 ==
  data: w input; q_dot_r output
function q_dot_r = ForwardKinematic(w)

r = 0.05 ; lx = 0.225 ; ly = 0.105 ;

Jacobian_T = (r/4) * [1, 1, 1, 1; 1, -1, 1, -1; -1/(lx + ly), 1/(lx + ly), 1/(lx + ly), -1/(lx + ly)];

q_dot_r = Jacobian_T * w;

== matlab function MobileSimulator/DesiresTrajectory ==
  data: t input; q output
function q  = Desired_Trajectory(t)
%Create desires trajectory

% Radius and vecolcity angular
R = 20 ;

% Parametric equation
%x_d = R*sin(t);
%y_d = R*cos(t);

x_d = 0 + 0.5*sin(100*t);
y_d = 0 + 0.5*cos(100*t);

% Derivative of Paramet ric equation
%x_dot_d = R*cos(t);
%y_dot_d = -R*sin(t);
x_dot_d = 0.1;
y_dot_d = 0.1;

theta_d = 0;

% Output
if (x_d >= 5)
    x_d = 5;
    y_d = 5;
end
q = [x_d; y_d; theta_d];

== matlab function MobileSimulator/ForwardKinematic ==
  data: w input; q_dot_r output
function q_dot_r = ForwardKinematic(w)

r = 0.03 ; lx = 0.1 ; ly = 0.075 ;

Jacobian_T = (r/4) * [1, 1, 1, 1; -1, 1, 1, -1; -1/(lx + ly), 1/(lx + ly), -1/(lx + ly), 1/(lx + ly)];

q_dot_r = Jacobian_T * w;

== matlab function MobileSimulator/ToGlobal ==
  data: q_r input; theta input; q output
function q = Transform(q_r, theta)

% This function to transform global coordinates to mobile platform coordinates

% Transform matrix
R = [cos(theta), -sin(theta), 0; sin(theta), cos(theta), 0; 0, 0, 1];


% Output
q = R * q_r;
